simulink model "LQRPosWithCMD"  (R2024a)
settings: Solver=VariableStepAuto  StartTime=0.0  StopTime=65  RelTol=1e-3
undefined symbols (not defined in the file): A_pos, B_pos, C_pos, lqrd, Qpsi_pos, Qx_pos, Qy_pos, Qz_pos, Ts, Vehicle
libraries: dspstat3 x3, simulink x1
settings Model: Creator=advay  LastModifiedBy=advay

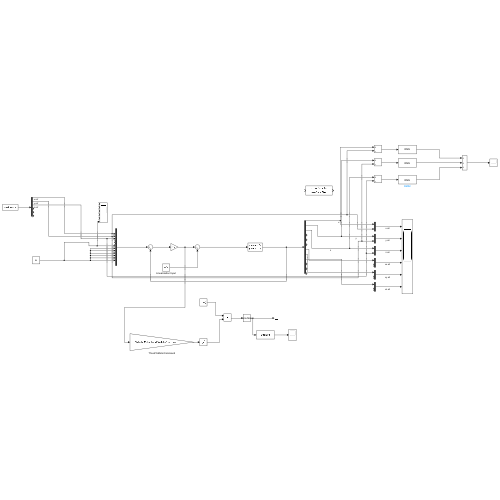
[thumbnail: Simulink's stored preview of the top-level diagram]
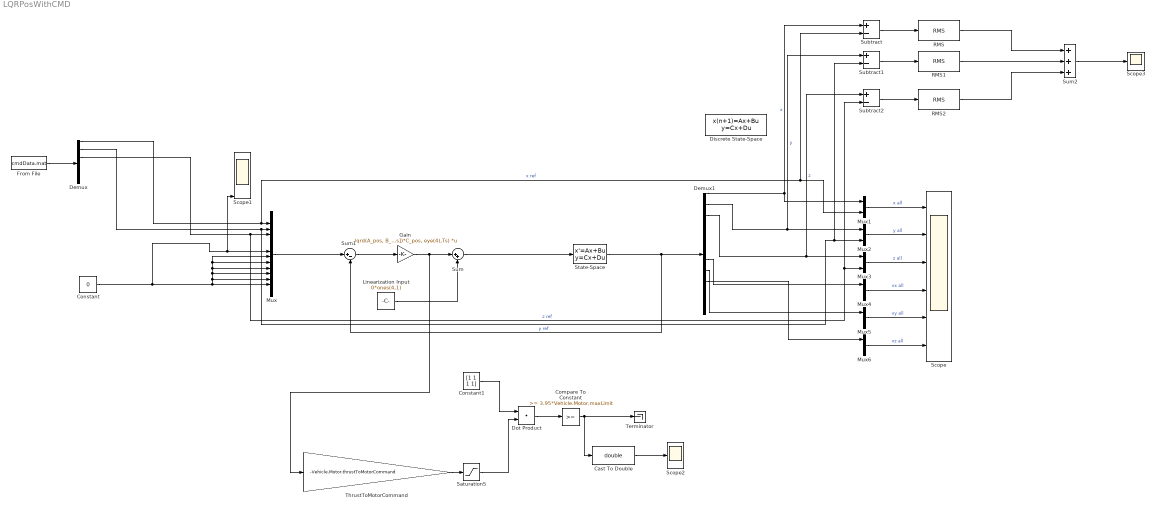
== system LQRPosWithCMD ==
  Cast To Double : DataTypeConversion  OutDataTypeStr=double  SaturateOnIntegerOverflow=off  RndMeth=Floor
  Compare To Constant : simulink/Logic and Bit Operations/Compare To Constant  relop=>=  const=3.95*Vehicle.Motor.maxLimit  OutDataTypeStr=boolean
  Constant : Constant  Value=0  SampleTime=Ts
  Constant1 : Constant  Value=[1 1 1 1]  OutDataTypeStr=double
  Demux : Demux  Outputs=6
  Demux1 : Demux  Outputs=12
  Discrete State-Space : DiscreteStateSpace  A=A_pos  B=B_pos  C=eye(12)  D=zeros(12,4)  SampleTime=Ts
  Dot Product : DotProduct  OutDataTypeStr=Inherit: Inherit via internal rule
  From File : FromFile  FileName=cmdData.mat  SampleTime=Ts
  Gain : Gain  Gain=lqrd(A_pos, B_pos, C_pos'*diag([Qx_pos, Qy_pos, Qz_pos, Qpsi_pos])*C_pos, eye(4),Ts)  Multiplication=Matrix(K*u)
  Linearization Input : Constant  Value=0*ones(4,1)  OutDataTypeStr=double  SampleTime=Ts
  Mux : Mux  Inputs=12
  Mux{1..6} (6 alike) : Mux  Inputs=2
  RMS : dspstat3/RMS  run=off  directionMode=Each column  dimension=1  InputProcessing=Columns as channels (frame based)  reset_popup=None
  RMS1 : dspstat3/RMS  run=off  directionMode=Each column  dimension=1  InputProcessing=Columns as channels (frame based)  reset_popup=None
  RMS2 : dspstat3/RMS  run=off  directionMode=Each column  dimension=1  InputProcessing=Columns as channels (frame based)  reset_popup=None
  Saturation5 : Saturate  UpperLimit=Vehicle.Motor.maxLimit  LowerLimit=Vehicle.Motor.minLimit
  Scope : Scope  NumInputPorts=6
  Scope1 : Scope  NumInputPorts=6
  Scope2 : Scope
  Scope3 : Scope
  State-Space : StateSpace  A=A_pos  B=B_pos  C=eye(12)  D=zeros(12,4)  InitialCondition=0
  Subtract : Sum  Inputs=+-
  Subtract1 : Sum  Inputs=+-
  Subtract2 : Sum  Inputs=+-
  Sum : Sum  Inputs=|++
  Sum1 : Sum  Inputs=|+-
  Sum2 : Sum  Inputs=+++
  Terminator : Terminator
  ThrustToMotorCommand : Gain  Gain=-Vehicle.Motor.thrustToMotorCommand
  wires:
  Gain/1 -> ThrustToMotorCommand/1, Sum/1
  Compare To Constant/1 -> Cast To Double/1, Terminator/1
  Constant/1 -> Scope1/6, Mux/6, Mux/12, Mux/11, Mux/10, Mux/9, Mux/8, Mux/7
  Sum/1 -> State-Space/1
  Constant1/1 -> Dot Product/1
  ThrustToMotorCommand/1 -> Saturation5/1
  Cast To Double/1 -> Scope2/1
  Mux3/1 -> Scope/3  "z all"
  Mux6/1 -> Scope/6  "vz all"
  Demux1/7 -> Mux4/1
  Demux1/8 -> Mux5/1
  Mux4/1 -> Scope/4  "vx all"
  Mux/1 -> Sum1/1
  Demux1/3 -> Subtract2/1, Mux3/1  "z"
  Demux1/2 -> Subtract1/1, Mux2/1  "y"
  State-Space/1 -> Sum1/2, Demux1/1
  Dot Product/1 -> Compare To Constant/1
  Demux1/1 -> Subtract/1, Mux1/1  "x"
  Mux1/1 -> Scope/1  "x all"
  Sum1/1 -> Gain/1
  Mux5/1 -> Scope/5  "vy all"
  Saturation5/1 -> Dot Product/2
  Mux2/1 -> Scope/2  "y all"
  Demux1/9 -> Mux6/1
  Linearization Input/1 -> Sum/2
  From File/1 -> Demux/1
  Demux/1 -> Mux1/2, Subtract/2, Mux/1  "x ref"
  Demux/2 -> Mux2/2, Subtract1/2, Mux/2  "y ref"
  Demux/3 -> Subtract2/2, Mux3/2, Mux/3  "z ref"
  Subtract/1 -> RMS/1
  Subtract1/1 -> RMS1/1
  Subtract2/1 -> RMS2/1
  RMS2/1 -> Sum2/3
  RMS/1 -> Sum2/1
  RMS1/1 -> Sum2/2
  Sum2/1 -> Scope3/1
